simulink model "SpeedControlTest_vDemo_TC"  (Simulink 6.6)
settings: Solver=ode4  SolverMode=SingleTasking  StartTime=0.0  StopTime=252  FixedStep=0.01  RelTol=1e-3
InitFcn:
  | tempomat_para
StopFcn:
  | clear;
values from neighbouring files (symbols this model uses):
  A = 1.9    [tempomat_para.m]
  a_Fzg_max = 2    [tempomat_para.m]
  a_Fzg_min = -2    [tempomat_para.m]
  cw = 0.32    [tempomat_para.m]
  gang = [1 2 3 4]    [tempomat_para.m]
  gang_vec = [1 2 3 4]    [tempomat_para.m]
  i_anteil = 5    [tempomat_para.m]
  i_d = 3.42    [tempomat_para.m]
  i_g = [3.91 2.17 1.37 1.00]    [tempomat_para.m]
  lambda_gang = [1.3 1.25  1.17  1.05]    [tempomat_para.m]
  m_Fzg = 1400    [tempomat_para.m]
  M_mot_max = [130 149 163 170 168 166 162 158 150 139 123 80]    [tempomat_para.m]
  M_mot_min = [0 -40]    [tempomat_para.m]
  n_mot0 = 1000    [tempomat_para.m]
  n_mot_max = 1000:500:6500    [tempomat_para.m]
  n_mot_min = [1000 6500]    [tempomat_para.m]
  p_anteil = 100    [tempomat_para.m]
  r_dyn = 0.28    [tempomat_para.m]
  rho = 1.202    [tempomat_para.m]
  t_sch = 0.2    [tempomat_para.m]
  TI = [block '/TI']    [PSTI_callback.m]
  v_Fzg_ms0 = 0    [tempomat_para.m]
undefined symbols (not defined in the file or in its folder): Drossel_mat, getdatatypespecs
libraries: simulink x113, fzgbib x3
(part 7 of 9)

== system SpeedControlTest_vDemo_TC/Validation Functions/R2 Speed Control velocity restoration time after simple  acceleration or deceleration/after (6 seconds)  |V_Des-V_Vhcl <= 1.4|/PAS1/none - pass - fail/Arbitration ==
  Pass : Inport
  Fail1 : Inport  Port=2
  Fail2 : Inport  Port=3
  Fail3 : Inport  Port=4
  Fail4 : Inport  Port=5
  Delay P F1 F3 : Inport  Port=6
  Delay F2 : Inport  Port=7
  Delay F4 : Inport  Port=8
  Max delay : Inport  Port=9
  Verdict identification : Subsystem
  Verdict selection : Subsystem
  Verdict : Outport
  Delay : Outport  Port=2
  wires:
  Verdict selection/2(Delay) -> Delay/1
  Verdict selection/1(Verdict) -> Verdict/1
  Max delay/1 -> Verdict selection/6(Max delay)
  Verdict identification/2(V2) -> Verdict selection/2(V2)
  Verdict identification/1(V1) -> Verdict selection/1(V1)
  Delay F4/1 -> Verdict selection/5(Delay F4)
  Delay F2/1 -> Verdict selection/4(Delay F2)
  Delay P F1 F3/1 -> Verdict selection/3(Delay P F1 F3)
  Fail4/1 -> Verdict identification/5(Fail4)
  Fail3/1 -> Verdict identification/4(Fail3)
  Fail2/1 -> Verdict identification/3(Fail2)
  Fail1/1 -> Verdict identification/2(Fail1)
  Pass/1 -> Verdict identification/1(Pass)

== system SpeedControlTest_vDemo_TC/Validation Functions/R2 Speed Control velocity restoration time after simple  acceleration or deceleration/after (6 seconds)  |V_Des-V_Vhcl <= 1.4|/PAS1/none - pass - fail/Compute delay ==
  Max Delay : Inport
  R AND : Inport  Port=2
  Clock : Clock
      settings: Decimation=10
  Clock1 : Clock
      settings: Decimation=10
  Divide : Product  Inputs=/*  OutScaling=2^-10
  Hold1 : Subsystem  TreatAsAtomicUnit=on
      mask Display: patch(-0.31+[0.4 0.46 0.46 0.54 0.54 0.6 0.6 0.55 0.55 0.45 0.45 0.4],-0.19+[0.85 0.85 0.95 0.95 0.85 0.85 0.87 0.87 0.96 0.96 0.87 0.87],[0 0 0]);
  SimStepSize : Constant  Value=0.01
  Subtract : Sum  Inputs=-+  OutScaling=2^-10
  Subtract1 : Sum  Inputs=+-  OutScaling=2^-10
  Delay : Outport
  wires:
  Divide/1 -> Delay/1
  Max Delay/1 -> Subtract/1
  SimStepSize/1 -> Divide/1
  Clock/1 -> Hold1/2("    ")
  Subtract/1 -> Subtract1/2
  Subtract1/1 -> Divide/2
  Clock1/1 -> Subtract1/1
  Hold1/1("  ") -> Subtract/2
  R AND/1 -> Hold1/1(" ")

== system SpeedControlTest_vDemo_TC/Validation Functions/R2 Speed Control velocity restoration time after simple  acceleration or deceleration/after (6 seconds)  |V_Des-V_Vhcl <= 1.4|/PAS1/none - pass - fail/Compute delay1 ==
  Max Delay : Inport
  R AND/z : Inport  Port=2
  Add : Sum  OutScaling=2^-10
  Clock : Clock
      settings: Decimation=10
  Clock1 : Clock
      settings: Decimation=10
  Divide : Product  Inputs=/*  OutScaling=2^-10
  Hold1 : Subsystem  TreatAsAtomicUnit=on
      mask Display: patch(-0.31+[0.4 0.46 0.46 0.54 0.54 0.6 0.6 0.55 0.55 0.45 0.45 0.4],-0.19+[0.85 0.85 0.95 0.95 0.85 0.85 0.87 0.87 0.96 0.96 0.87 0.87],[0 0 0]);
  SimStepSize : Constant  Value=0.01
  Subtract : Sum  Inputs=-+  OutScaling=2^-10
  Subtract1 : Sum  Inputs=+-  OutScaling=2^-10
  Unit : Constant
  Delay : Outport
  wires:
  Divide/1 -> Add/2
  Unit/1 -> Add/1
  Max Delay/1 -> Subtract/1
  SimStepSize/1 -> Divide/1
  Clock/1 -> Hold1/2("    ")
  Subtract/1 -> Subtract1/2
  Subtract1/1 -> Divide/2
  Clock1/1 -> Subtract1/1
  Hold1/1("  ") -> Subtract/2
  R AND/z/1 -> Hold1/1(" ")
  Add/1 -> Delay/1

== system SpeedControlTest_vDemo_TC/Validation Functions/R2 Speed Control velocity restoration time after simple  acceleration or deceleration/after (6 seconds)  |V_Des-V_Vhcl <= 1.4|/PAS1/none - pass - fail/Compute delay2 ==
  Max Delay : Inport
  Rp & NOT(Ra) : Inport  Port=2
  Clock : Clock
      settings: Decimation=10
  Clock1 : Clock
      settings: Decimation=10
  Divide : Product  Inputs=/*  OutScaling=2^-10
  Hold1 : Subsystem  TreatAsAtomicUnit=on
      mask Display: patch(-0.31+[0.4 0.46 0.46 0.54 0.54 0.6 0.6 0.55 0.55 0.45 0.45 0.4],-0.19+[0.85 0.85 0.95 0.95 0.85 0.85 0.87 0.87 0.96 0.96 0.87 0.87],[0 0 0]);
  SimStepSize : Constant  Value=0.01
  Subtract : Sum  Inputs=-+  OutScaling=2^-10
  Subtract1 : Sum  Inputs=+-  OutScaling=2^-10
  Delay : Outport
  wires:
  Divide/1 -> Delay/1
  Rp & NOT(Ra)/1 -> Hold1/1(" ")
  Hold1/1("  ") -> Subtract/2
  Clock1/1 -> Subtract1/1
  Subtract1/1 -> Divide/2
  Subtract/1 -> Subtract1/2
  Clock/1 -> Hold1/2("    ")
  SimStepSize/1 -> Divide/1
  Max Delay/1 -> Subtract/1

== system SpeedControlTest_vDemo_TC/Validation Functions/R2 Speed Control velocity restoration time after simple  acceleration or deceleration/after (6 seconds)  |V_Des-V_Vhcl <= 1.4|/PAS1/none - pass - fail/Hold R AND1 ==
  " " : Inport
  "    " : Inport  Port=2
  Memory : Memory  Orientation=left
  Switch : Switch  Criteria=u2 ~= 0
  "  " : Outport
  wires:
  Memory/1 -> Switch/3
  Switch/1 -> Memory/1, "  "/1
  "    "/1 -> Switch/1
  " "/1 -> Switch/2

== system SpeedControlTest_vDemo_TC/Validation Functions/R2 Speed Control velocity restoration time after simple  acceleration or deceleration/after (6 seconds)  |V_Des-V_Vhcl <= 1.4|/PAS1/none - pass - fail/Hold R AND2 ==
  " " : Inport
  "    " : Inport  Port=2
  Memory : Memory  Orientation=left
  Switch : Switch  Criteria=u2 ~= 0
  "  " : Outport
  wires:
  Memory/1 -> Switch/3
  Switch/1 -> Memory/1, "  "/1
  "    "/1 -> Switch/1
  " "/1 -> Switch/2

== system SpeedControlTest_vDemo_TC/Validation Functions/R2 Speed Control velocity restoration time after simple  acceleration or deceleration/after (6 seconds)  |V_Des-V_Vhcl <= 1.4|/PAS1/none - pass - fail/Hold R AND3 ==
  " " : Inport
  "    " : Inport  Port=2
  Memory : Memory  Orientation=left
  Switch : Switch  Criteria=u2 ~= 0
  "  " : Outport
  wires:
  " "/1 -> Switch/2
  "    "/1 -> Switch/1
  Switch/1 -> "  "/1, Memory/1
  Memory/1 -> Switch/3

== system SpeedControlTest_vDemo_TC/Validation Functions/R2 Speed Control velocity restoration time after simple  acceleration or deceleration/after (6 seconds)  |V_Des-V_Vhcl <= 1.4|/PAS1/none - pass - fail/Hold1 ==
  " " : Inport
  "    " : Inport  Port=2
  Memory : Memory  Orientation=left
  Switch : Switch  Criteria=u2 ~= 0
  "  " : Outport
  wires:
  Memory/1 -> Switch/3
  Switch/1 -> Memory/1, "  "/1
  "    "/1 -> Switch/1
  " "/1 -> Switch/2

== system SpeedControlTest_vDemo_TC/Validation Functions/R2 Speed Control velocity restoration time after simple  acceleration or deceleration/after (6 seconds)  |V_Des-V_Vhcl <= 1.4|/PAS1/none - pass - fail/Hold2 ==
  " " : Inport
  "    " : Inport  Port=2
  Memory : Memory  Orientation=left
  Switch : Switch  Criteria=u2 ~= 0
  "  " : Outport
  wires:
  Memory/1 -> Switch/3
  Switch/1 -> Memory/1, "  "/1
  "    "/1 -> Switch/1
  " "/1 -> Switch/2

== system SpeedControlTest_vDemo_TC/Validation Functions/R2 Speed Control velocity restoration time after simple  acceleration or deceleration/after (6 seconds)  |V_Des-V_Vhcl <= 1.4|/PAS1/none - pass - fail/Hold3 ==
  " " : Inport
  "    " : Inport  Port=2
  Memory : Memory  Orientation=left
  Switch : Switch  Criteria=u2 ~= 0
  "  " : Outport
  wires:
  " "/1 -> Switch/2
  "    "/1 -> Switch/1
  Switch/1 -> "  "/1, Memory/1
  Memory/1 -> Switch/3

== system SpeedControlTest_vDemo_TC/Validation Functions/R2 Speed Control velocity restoration time after simple  acceleration or deceleration/after (6 seconds)  |V_Des-V_Vhcl <= 1.4|/PAS1/none - pass - fail/Hold4 ==
  " " : Inport
  "    " : Inport  Port=2
  Memory : Memory  Orientation=left
  Switch : Switch  Criteria=u2 ~= 0
  "  " : Outport
  wires:
  Memory/1 -> Switch/3
  Switch/1 -> Memory/1, "  "/1
  "    "/1 -> Switch/1
  " "/1 -> Switch/2

== system SpeedControlTest_vDemo_TC/Validation Functions/R2 Speed Control velocity restoration time after simple  acceleration or deceleration/after (6 seconds)  |V_Des-V_Vhcl <= 1.4|/PAS1/none - pass - fail/Hold5 ==
  " " : Inport
  "    " : Inport  Port=2
  Memory : Memory  Orientation=left
  Switch : Switch  Criteria=u2 ~= 0
  "  " : Outport
  wires:
  " "/1 -> Switch/2
  "    "/1 -> Switch/1
  Switch/1 -> "  "/1, Memory/1
  Memory/1 -> Switch/3

== system SpeedControlTest_vDemo_TC/Validation Functions/R2 Speed Control velocity restoration time after simple  acceleration or deceleration/after (6 seconds)  |V_Des-V_Vhcl <= 1.4|/PAS2/Delay bus signals/AD delay ==
  In1 : Inport
  Delay : Constant  Value=0
  Integer Delay : S-Function  FunctionName=sfix_udelay  Parameters=samptime,vinit,NumDelays,1,1,0  mask(Integer Delay){vinit=0.0, samptime=-1, NumDelays=15}
      mask prompts: vinit "Initial condition:"; samptime "Sample time:"; NumDelays "Number of delays:"
      mask help: Delay a signal N sample periods.
      mask init:
      | if isempty(NumDelays)
      |    NumDelays = 1;
      | end
      mask Display: fprintf(' %d\nZ   ',-1*(NumDelays))
  Switch : Switch  Criteria=u2 ~= 0
  Out1 : Outport
  wires:
  Switch/1 -> Out1/1
  In1/1 -> Switch/3, Integer Delay/1
  Delay/1 -> Switch/2
  Integer Delay/1 -> Switch/1

== system SpeedControlTest_vDemo_TC/Validation Functions/R2 Speed Control velocity restoration time after simple  acceleration or deceleration/after (6 seconds)  |V_Des-V_Vhcl <= 1.4|/PAS2/Delay bus signals/ELL delay ==
  In1 : Inport
  Delay : Constant  Value=0
  Integer Delay : S-Function  FunctionName=sfix_udelay  Parameters=samptime,vinit,NumDelays,1,1,0  mask(Integer Delay){vinit=0.0, samptime=-1, NumDelays=15}
      mask prompts: vinit "Initial condition:"; samptime "Sample time:"; NumDelays "Number of delays:"
      mask help: Delay a signal N sample periods.
      mask init:
      | if isempty(NumDelays)
      |    NumDelays = 1;
      | end
      mask Display: fprintf(' %d\nZ   ',-1*(NumDelays))
  Switch : Switch  Criteria=u2 ~= 0
  Out1 : Outport
  wires:
  Switch/1 -> Out1/1
  In1/1 -> Switch/3, Integer Delay/1
  Delay/1 -> Switch/2
  Integer Delay/1 -> Switch/1

== system SpeedControlTest_vDemo_TC/Validation Functions/R2 Speed Control velocity restoration time after simple  acceleration or deceleration/after (6 seconds)  |V_Des-V_Vhcl <= 1.4|/PAS2/Delay bus signals/EUL delay ==
  In1 : Inport
  Delay : Constant  Value=0
  Integer Delay : S-Function  FunctionName=sfix_udelay  Parameters=samptime,vinit,NumDelays,1,1,0  mask(Integer Delay){vinit=0.0, samptime=-1, NumDelays=15}
      mask prompts: vinit "Initial condition:"; samptime "Sample time:"; NumDelays "Number of delays:"
      mask help: Delay a signal N sample periods.
      mask init:
      | if isempty(NumDelays)
      |    NumDelays = 1;
      | end
      mask Display: fprintf(' %d\nZ   ',-1*(NumDelays))
  Switch : Switch  Criteria=u2 ~= 0
  Out1 : Outport
  wires:
  Integer Delay/1 -> Switch/1
  Delay/1 -> Switch/2
  In1/1 -> Integer Delay/1, Switch/3
  Switch/1 -> Out1/1

== system SpeedControlTest_vDemo_TC/Validation Functions/R2 Speed Control velocity restoration time after simple  acceleration or deceleration/after (6 seconds)  |V_Des-V_Vhcl <= 1.4|/PAS2/none - pass - fail/Arbitration ==
  Pass : Inport
  Fail1 : Inport  Port=2
  Fail2 : Inport  Port=3
  Fail3 : Inport  Port=4
  Fail4 : Inport  Port=5
  Delay P F1 F3 : Inport  Port=6
  Delay F2 : Inport  Port=7
  Delay F4 : Inport  Port=8
  Max delay : Inport  Port=9
  Verdict identification : Subsystem
  Verdict selection : Subsystem
  Verdict : Outport
  Delay : Outport  Port=2
  wires:
  Verdict selection/2(Delay) -> Delay/1
  Verdict selection/1(Verdict) -> Verdict/1
  Max delay/1 -> Verdict selection/6(Max delay)
  Verdict identification/2(V2) -> Verdict selection/2(V2)
  Verdict identification/1(V1) -> Verdict selection/1(V1)
  Delay F4/1 -> Verdict selection/5(Delay F4)
  Delay F2/1 -> Verdict selection/4(Delay F2)
  Delay P F1 F3/1 -> Verdict selection/3(Delay P F1 F3)
  Fail4/1 -> Verdict identification/5(Fail4)
  Fail3/1 -> Verdict identification/4(Fail3)
  Fail2/1 -> Verdict identification/3(Fail2)
  Fail1/1 -> Verdict identification/2(Fail1)
  Pass/1 -> Verdict identification/1(Pass)

== system SpeedControlTest_vDemo_TC/Validation Functions/R2 Speed Control velocity restoration time after simple  acceleration or deceleration/after (6 seconds)  |V_Des-V_Vhcl <= 1.4|/PAS2/none - pass - fail/Compute delay ==
  Max Delay : Inport
  R AND : Inport  Port=2
  Clock : Clock
      settings: Decimation=10
  Clock1 : Clock
      settings: Decimation=10
  Divide : Product  Inputs=/*  OutScaling=2^-10
  Hold1 : Subsystem  TreatAsAtomicUnit=on
      mask Display: patch(-0.31+[0.4 0.46 0.46 0.54 0.54 0.6 0.6 0.55 0.55 0.45 0.45 0.4],-0.19+[0.85 0.85 0.95 0.95 0.85 0.85 0.87 0.87 0.96 0.96 0.87 0.87],[0 0 0]);
  SimStepSize : Constant  Value=0.01
  Subtract : Sum  Inputs=-+  OutScaling=2^-10
  Subtract1 : Sum  Inputs=+-  OutScaling=2^-10
  Delay : Outport
  wires:
  Divide/1 -> Delay/1
  Max Delay/1 -> Subtract/1
  SimStepSize/1 -> Divide/1
  Clock/1 -> Hold1/2("    ")
  Subtract/1 -> Subtract1/2
  Subtract1/1 -> Divide/2
  Clock1/1 -> Subtract1/1
  Hold1/1("  ") -> Subtract/2
  R AND/1 -> Hold1/1(" ")

== system SpeedControlTest_vDemo_TC/Validation Functions/R2 Speed Control velocity restoration time after simple  acceleration or deceleration/after (6 seconds)  |V_Des-V_Vhcl <= 1.4|/PAS2/none - pass - fail/Compute delay1 ==
  Max Delay : Inport
  R AND/z : Inport  Port=2
  Add : Sum  OutScaling=2^-10
  Clock : Clock
      settings: Decimation=10
  Clock1 : Clock
      settings: Decimation=10
  Divide : Product  Inputs=/*  OutScaling=2^-10
  Hold1 : Subsystem  TreatAsAtomicUnit=on
      mask Display: patch(-0.31+[0.4 0.46 0.46 0.54 0.54 0.6 0.6 0.55 0.55 0.45 0.45 0.4],-0.19+[0.85 0.85 0.95 0.95 0.85 0.85 0.87 0.87 0.96 0.96 0.87 0.87],[0 0 0]);
  SimStepSize : Constant  Value=0.01
  Subtract : Sum  Inputs=-+  OutScaling=2^-10
  Subtract1 : Sum  Inputs=+-  OutScaling=2^-10
  Unit : Constant
  Delay : Outport
  wires:
  Divide/1 -> Add/2
  Unit/1 -> Add/1
  Max Delay/1 -> Subtract/1
  SimStepSize/1 -> Divide/1
  Clock/1 -> Hold1/2("    ")
  Subtract/1 -> Subtract1/2
  Subtract1/1 -> Divide/2
  Clock1/1 -> Subtract1/1
  Hold1/1("  ") -> Subtract/2
  R AND/z/1 -> Hold1/1(" ")
  Add/1 -> Delay/1

== system SpeedControlTest_vDemo_TC/Validation Functions/R2 Speed Control velocity restoration time after simple  acceleration or deceleration/after (6 seconds)  |V_Des-V_Vhcl <= 1.4|/PAS2/none - pass - fail/Compute delay2 ==
  Max Delay : Inport
  Rp & NOT(Ra) : Inport  Port=2
  Clock : Clock
      settings: Decimation=10
  Clock1 : Clock
      settings: Decimation=10
  Divide : Product  Inputs=/*  OutScaling=2^-10
  Hold1 : Subsystem  TreatAsAtomicUnit=on
      mask Display: patch(-0.31+[0.4 0.46 0.46 0.54 0.54 0.6 0.6 0.55 0.55 0.45 0.45 0.4],-0.19+[0.85 0.85 0.95 0.95 0.85 0.85 0.87 0.87 0.96 0.96 0.87 0.87],[0 0 0]);
  SimStepSize : Constant  Value=0.01
  Subtract : Sum  Inputs=-+  OutScaling=2^-10
  Subtract1 : Sum  Inputs=+-  OutScaling=2^-10
  Delay : Outport
  wires:
  Divide/1 -> Delay/1
  Rp & NOT(Ra)/1 -> Hold1/1(" ")
  Hold1/1("  ") -> Subtract/2
  Clock1/1 -> Subtract1/1
  Subtract1/1 -> Divide/2
  Subtract/1 -> Subtract1/2
  Clock/1 -> Hold1/2("    ")
  SimStepSize/1 -> Divide/1
  Max Delay/1 -> Subtract/1

== system SpeedControlTest_vDemo_TC/Validation Functions/R2 Speed Control velocity restoration time after simple  acceleration or deceleration/after (6 seconds)  |V_Des-V_Vhcl <= 1.4|/PAS2/none - pass - fail/Hold R AND1 ==
  " " : Inport
  "    " : Inport  Port=2
  Memory : Memory  Orientation=left
  Switch : Switch  Criteria=u2 ~= 0
  "  " : Outport
  wires:
  Memory/1 -> Switch/3
  Switch/1 -> Memory/1, "  "/1
  "    "/1 -> Switch/1
  " "/1 -> Switch/2

== system SpeedControlTest_vDemo_TC/Validation Functions/R2 Speed Control velocity restoration time after simple  acceleration or deceleration/after (6 seconds)  |V_Des-V_Vhcl <= 1.4|/PAS2/none - pass - fail/Hold R AND2 ==
  " " : Inport
  "    " : Inport  Port=2
  Memory : Memory  Orientation=left
  Switch : Switch  Criteria=u2 ~= 0
  "  " : Outport
  wires:
  Memory/1 -> Switch/3
  Switch/1 -> Memory/1, "  "/1
  "    "/1 -> Switch/1
  " "/1 -> Switch/2

== system SpeedControlTest_vDemo_TC/Validation Functions/R2 Speed Control velocity restoration time after simple  acceleration or deceleration/after (6 seconds)  |V_Des-V_Vhcl <= 1.4|/PAS2/none - pass - fail/Hold R AND3 ==
  " " : Inport
  "    " : Inport  Port=2
  Memory : Memory  Orientation=left
  Switch : Switch  Criteria=u2 ~= 0
  "  " : Outport
  wires:
  " "/1 -> Switch/2
  "    "/1 -> Switch/1
  Switch/1 -> "  "/1, Memory/1
  Memory/1 -> Switch/3

== system SpeedControlTest_vDemo_TC/Validation Functions/R2 Speed Control velocity restoration time after simple  acceleration or deceleration/after (6 seconds)  |V_Des-V_Vhcl <= 1.4|/PAS2/none - pass - fail/Hold1 ==
  " " : Inport
  "    " : Inport  Port=2
  Memory : Memory  Orientation=left
  Switch : Switch  Criteria=u2 ~= 0
  "  " : Outport
  wires:
  Memory/1 -> Switch/3
  Switch/1 -> Memory/1, "  "/1
  "    "/1 -> Switch/1
  " "/1 -> Switch/2

== system SpeedControlTest_vDemo_TC/Validation Functions/R2 Speed Control velocity restoration time after simple  acceleration or deceleration/after (6 seconds)  |V_Des-V_Vhcl <= 1.4|/PAS2/none - pass - fail/Hold2 ==
  " " : Inport
  "    " : Inport  Port=2
  Memory : Memory  Orientation=left
  Switch : Switch  Criteria=u2 ~= 0
  "  " : Outport
  wires:
  Memory/1 -> Switch/3
  Switch/1 -> Memory/1, "  "/1
  "    "/1 -> Switch/1
  " "/1 -> Switch/2

== system SpeedControlTest_vDemo_TC/Validation Functions/R2 Speed Control velocity restoration time after simple  acceleration or deceleration/after (6 seconds)  |V_Des-V_Vhcl <= 1.4|/PAS2/none - pass - fail/Hold3 ==
  " " : Inport
  "    " : Inport  Port=2
  Memory : Memory  Orientation=left
  Switch : Switch  Criteria=u2 ~= 0
  "  " : Outport
  wires:
  " "/1 -> Switch/2
  "    "/1 -> Switch/1
  Switch/1 -> "  "/1, Memory/1
  Memory/1 -> Switch/3

== system SpeedControlTest_vDemo_TC/Validation Functions/R2 Speed Control velocity restoration time after simple  acceleration or deceleration/after (6 seconds)  |V_Des-V_Vhcl <= 1.4|/PAS2/none - pass - fail/Hold4 ==
  " " : Inport
  "    " : Inport  Port=2
  Memory : Memory  Orientation=left
  Switch : Switch  Criteria=u2 ~= 0
  "  " : Outport
  wires:
  Memory/1 -> Switch/3
  Switch/1 -> Memory/1, "  "/1
  "    "/1 -> Switch/1
  " "/1 -> Switch/2

== system SpeedControlTest_vDemo_TC/Validation Functions/R2 Speed Control velocity restoration time after simple  acceleration or deceleration/after (6 seconds)  |V_Des-V_Vhcl <= 1.4|/PAS2/none - pass - fail/Hold5 ==
  " " : Inport
  "    " : Inport  Port=2
  Memory : Memory  Orientation=left
  Switch : Switch  Criteria=u2 ~= 0
  "  " : Outport
  wires:
  " "/1 -> Switch/2
  "    "/1 -> Switch/1
  Switch/1 -> "  "/1, Memory/1
  Memory/1 -> Switch/3

== system SpeedControlTest_vDemo_TC/Validation Functions/R2 Speed Control velocity restoration time after simple  acceleration or deceleration/after (6 seconds)  |V_Des-V_Vhcl <= 1.4|/R = 2/Active for  6s after R=1 /Time since R = 1 ==
  Signal : Inport
  Clock : Clock
      settings: Decimation=10
  Logical Operator : Logic  Operator=NAND  AllPortsSameDT=off  OutDataTypeMode=Boolean
  Logical Operator1 : Logic  Operator=NOT  AllPortsSameDT=off  OutDataTypeMode=Boolean
  Memory : Memory  Orientation=left
  Memory1 : Memory
  R = 1 : Subsystem
  Subtract : Sum  Inputs=-+  OutScaling=2^-10
  Switch : Switch  Criteria=u2 > Threshold
  Trigger : Outport
  Feature : Outport  Port=2
  wires:
  Logical Operator/1 -> Switch/2
  Logical Operator1/1 -> Logical Operator/2
  Memory1/1 -> Logical Operator1/1
  Memory/1 -> Switch/1
  Switch/1 -> Memory/1, Subtract/1
  Clock/1 -> Switch/3, Subtract/2
  Subtract/1 -> Feature/1
  R = 1/1(Out1) -> Memory1/1, Logical Operator/1, Trigger/1
  Signal/1 -> R = 1/1(In1)

== system SpeedControlTest_vDemo_TC/Validation Functions/R1 Speed Control step response/Complete step & CC active + no target & Speed Control active/Complete step detection/Step detection/Active if signals constant for some specified time/Time since signal constant ==
  Signal : Inport
  Clock : Clock
      settings: Decimation=10
  Detect constant : Subsystem  TreatAsAtomicUnit=on  mask(Feature extraction block){RT=0.001}
      mask prompts: RT "Relative tolerance in %"
      mask help: Detect if the signal value is constant (using the last two signal values) allowing for a user-defined relative deviation
      mask CallbackString:
      | if or( (str2double(get_param(gcb,'RT')) < 0), (str2double(get_param(gcb,'RT')) > 100))
      |     error(['Relative tolerance value (' get_param(gcb,'RT') ') out of range. Please give a value between 0 and 100.']);
      | else
      |     set_param([gcb '/Relative tolerance/Relative Tolerance'],'Value',get_param(gcb,'RT'));
      | end
  Logical Operator : Logic  Operator=NAND  AllPortsSameDT=off  OutDataTypeMode=Boolean
  Logical Operator1 : Logic  Operator=NOT  AllPortsSameDT=off  OutDataTypeMode=Boolean
  Memory : Memory  Orientation=left
  Memory1 : Memory
  Subtract : Sum  Inputs=-+  OutScaling=2^-10
  Switch : Switch  Criteria=u2 > Threshold
  Trigger : Outport
  Feature : Outport  Port=2
  wires:
  Logical Operator/1 -> Switch/2
  Logical Operator1/1 -> Logical Operator/2
  Memory1/1 -> Logical Operator1/1
  Memory/1 -> Switch/1
  Switch/1 -> Memory/1, Subtract/1
  Clock/1 -> Switch/3, Subtract/2
  Subtract/1 -> Feature/1
  Detect constant/1(Constant) -> Memory1/1, Logical Operator/1, Trigger/1
  Signal/1 -> Detect constant/1(Signal)

== system SpeedControlTest_vDemo_TC/Validation Functions/R1 Speed Control step response/Complete step & CC active + no target & Speed Control active/Complete step detection/Step detection/Active if signals constant for some specified time/Time since signal constant1 ==
  Signal : Inport
  Clock : Clock
      settings: Decimation=10
  Detect constant : Subsystem  TreatAsAtomicUnit=on  mask(Feature extraction block){RT=0.001}
      mask prompts: RT "Relative tolerance in %"
      mask help: Detect if the signal value is constant (using the last two signal values) allowing for a user-defined relative deviation
      mask CallbackString:
      | if or( (str2double(get_param(gcb,'RT')) < 0), (str2double(get_param(gcb,'RT')) > 100))
      |     error(['Relative tolerance value (' get_param(gcb,'RT') ') out of range. Please give a value between 0 and 100.']);
      | else
      |     set_param([gcb '/Relative tolerance/Relative Tolerance'],'Value',get_param(gcb,'RT'));
      | end
  Logical Operator : Logic  Operator=NAND  AllPortsSameDT=off  OutDataTypeMode=Boolean
  Logical Operator1 : Logic  Operator=NOT  AllPortsSameDT=off  OutDataTypeMode=Boolean
  Memory : Memory  Orientation=left
  Memory1 : Memory
  Subtract : Sum  Inputs=-+  OutScaling=2^-10
  Switch : Switch  Criteria=u2 > Threshold
  Trigger : Outport
  Feature : Outport  Port=2
  wires:
  Signal/1 -> Detect constant/1(Signal)
  Detect constant/1(Constant) -> Trigger/1, Logical Operator/1, Memory1/1
  Subtract/1 -> Feature/1
  Clock/1 -> Subtract/2, Switch/3
  Switch/1 -> Subtract/1, Memory/1
  Memory/1 -> Switch/1
  Memory1/1 -> Logical Operator1/1
  Logical Operator1/1 -> Logical Operator/2
  Logical Operator/1 -> Switch/2

== system SpeedControlTest_vDemo_TC/Validation Functions/R1 Speed Control step response/Complete step & CC active + no target & Speed Control active/Complete step detection/Step detection/Detect constant/Relative tolerance ==
  sig : Inport
  ref : Inport  Port=2
  Abs : Abs
  Abs1 : Abs
  Add : Sum  Inputs=+-  OutScaling=2^-10
  Divide1 : Product  Inputs=**/  OutScaling=2^-10
  Max : Constant  Value=100
  Relational Operator : RelationalOperator  Operator=<=  LogicOutDataTypeMode=Boolean
  Relative Tolerance : Constant  Value=0.0001
  sig == ref : Outport
  wires:
  Abs/1 -> Relational Operator/1
  Add/1 -> Abs/1
  sig/1 -> Add/1
  ref/1 -> Add/2, Abs1/1
  Divide1/1 -> Relational Operator/2
  Max/1 -> Divide1/3
  Relative Tolerance/1 -> Divide1/2
  Relational Operator/1 -> sig == ref/1
  Abs1/1 -> Divide1/1

== system SpeedControlTest_vDemo_TC/Validation Functions/R1 Speed Control step response/Complete step & CC active + no target & Speed Control active/Complete step detection/Step detection reset/Active if signals constant for some specified time/Time since signal constant ==
  Signal : Inport
  Clock : Clock
      settings: Decimation=10
  Detect constant : Subsystem  TreatAsAtomicUnit=on  mask(Feature extraction block){RT=0.0001}
      mask prompts: RT "Relative tolerance in %"
      mask help: Detect if the signal value is constant (using the last two signal values) allowing for a user-defined relative deviation
      mask CallbackString:
      | if or( (str2double(get_param(gcb,'RT')) < 0), (str2double(get_param(gcb,'RT')) > 100))
      |     error(['Relative tolerance value (' get_param(gcb,'RT') ') out of range. Please give a value between 0 and 100.']);
      | else
      |     set_param([gcb '/Relative tolerance/Relative Tolerance'],'Value',get_param(gcb,'RT'));
      | end
  Logical Operator : Logic  Operator=NAND  AllPortsSameDT=off  OutDataTypeMode=Boolean
  Logical Operator1 : Logic  Operator=NOT  AllPortsSameDT=off  OutDataTypeMode=Boolean
  Memory : Memory  Orientation=left
  Memory1 : Memory
  Subtract : Sum  Inputs=-+  OutScaling=2^-10
  Switch : Switch  Criteria=u2 > Threshold
  Trigger : Outport
  Feature : Outport  Port=2
  wires:
  Signal/1 -> Detect constant/1(Signal)
  Detect constant/1(Constant) -> Trigger/1, Logical Operator/1, Memory1/1
  Subtract/1 -> Feature/1
  Clock/1 -> Subtract/2, Switch/3
  Switch/1 -> Subtract/1, Memory/1
  Memory/1 -> Switch/1
  Memory1/1 -> Logical Operator1/1
  Logical Operator1/1 -> Logical Operator/2
  Logical Operator/1 -> Switch/2

== system SpeedControlTest_vDemo_TC/Validation Functions/R1 Speed Control step response/Complete step & CC active + no target & Speed Control active/Complete step detection/Step detection reset/Active if signals constant for some specified time/Time since signal constant1 ==
  Signal : Inport
  Clock : Clock
      settings: Decimation=10
  Detect constant : Subsystem  TreatAsAtomicUnit=on  mask(Feature extraction block){RT=0.0001}
      mask prompts: RT "Relative tolerance in %"
      mask help: Detect if the signal value is constant (using the last two signal values) allowing for a user-defined relative deviation
      mask CallbackString:
      | if or( (str2double(get_param(gcb,'RT')) < 0), (str2double(get_param(gcb,'RT')) > 100))
      |     error(['Relative tolerance value (' get_param(gcb,'RT') ') out of range. Please give a value between 0 and 100.']);
      | else
      |     set_param([gcb '/Relative tolerance/Relative Tolerance'],'Value',get_param(gcb,'RT'));
      | end
  Logical Operator : Logic  Operator=NAND  AllPortsSameDT=off  OutDataTypeMode=Boolean
  Logical Operator1 : Logic  Operator=NOT  AllPortsSameDT=off  OutDataTypeMode=Boolean
  Memory : Memory  Orientation=left
  Memory1 : Memory
  Subtract : Sum  Inputs=-+  OutScaling=2^-10
  Switch : Switch  Criteria=u2 > Threshold
  Trigger : Outport
  Feature : Outport  Port=2
  wires:
  Logical Operator/1 -> Switch/2
  Logical Operator1/1 -> Logical Operator/2
  Memory1/1 -> Logical Operator1/1
  Memory/1 -> Switch/1
  Switch/1 -> Memory/1, Subtract/1
  Clock/1 -> Switch/3, Subtract/2
  Subtract/1 -> Feature/1
  Detect constant/1(Constant) -> Memory1/1, Logical Operator/1, Trigger/1
  Signal/1 -> Detect constant/1(Signal)

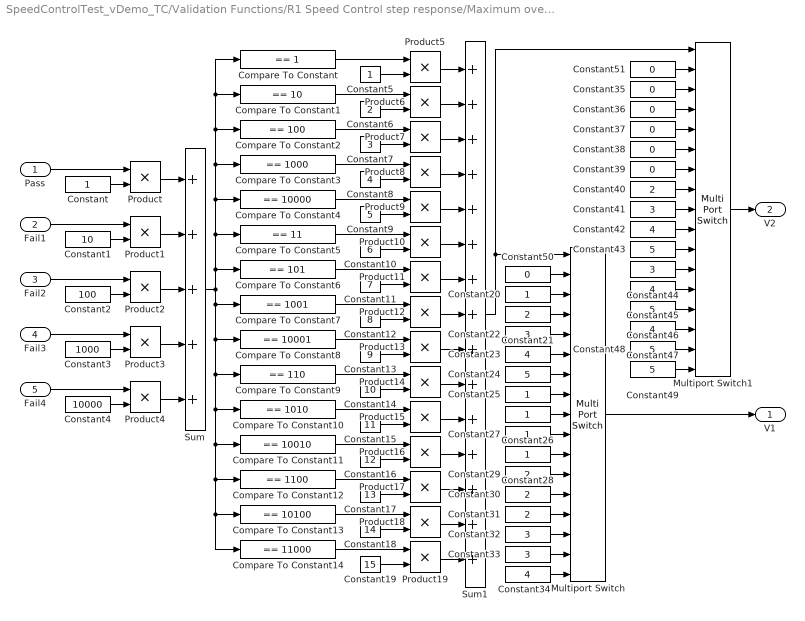
== system SpeedControlTest_vDemo_TC/Validation Functions/R1 Speed Control step response/Maximum overshoot < 5 &  Steady state error < 5/PAS/none - pass - fail/Arbitration/Verdict identification ==
  Pass : Inport
  Fail1 : Inport  Port=2
  Fail2 : Inport  Port=3
  Fail3 : Inport  Port=4
  Fail4 : Inport  Port=5
  Compare To Constant : simulink/Logic and Bit Operations/Compare To Constant  SystemSampleTime=-1  relop===  const=1  LogicOutDataTypeMode=uint8  ZeroCross=off
  Compare To Constant1 : simulink/Logic and Bit Operations/Compare To Constant  SystemSampleTime=-1  relop===  const=10  LogicOutDataTypeMode=uint8  ZeroCross=off
  Compare To Constant10 : simulink/Logic and Bit Operations/Compare To Constant  SystemSampleTime=-1  relop===  const=1010  LogicOutDataTypeMode=uint8  ZeroCross=off
  Compare To Constant11 : simulink/Logic and Bit Operations/Compare To Constant  SystemSampleTime=-1  relop===  const=10010  LogicOutDataTypeMode=uint8  ZeroCross=off
  Compare To Constant12 : simulink/Logic and Bit Operations/Compare To Constant  SystemSampleTime=-1  relop===  const=1100  LogicOutDataTypeMode=uint8  ZeroCross=off
  Compare To Constant13 : simulink/Logic and Bit Operations/Compare To Constant  SystemSampleTime=-1  relop===  const=10100  LogicOutDataTypeMode=uint8  ZeroCross=off
  Compare To Constant14 : simulink/Logic and Bit Operations/Compare To Constant  SystemSampleTime=-1  relop===  const=11000  LogicOutDataTypeMode=uint8  ZeroCross=off
  Compare To Constant2 : simulink/Logic and Bit Operations/Compare To Constant  SystemSampleTime=-1  relop===  const=100  LogicOutDataTypeMode=uint8  ZeroCross=off
  Compare To Constant3 : simulink/Logic and Bit Operations/Compare To Constant  SystemSampleTime=-1  relop===  const=1000  LogicOutDataTypeMode=uint8  ZeroCross=off
  Compare To Constant4 : simulink/Logic and Bit Operations/Compare To Constant  SystemSampleTime=-1  relop===  const=10000  LogicOutDataTypeMode=uint8  ZeroCross=off
  Compare To Constant5 : simulink/Logic and Bit Operations/Compare To Constant  SystemSampleTime=-1  relop===  const=11  LogicOutDataTypeMode=uint8  ZeroCross=off
  Compare To Constant6 : simulink/Logic and Bit Operations/Compare To Constant  SystemSampleTime=-1  relop===  const=101  LogicOutDataTypeMode=uint8  ZeroCross=off
  Compare To Constant7 : simulink/Logic and Bit Operations/Compare To Constant  SystemSampleTime=-1  relop===  const=1001  LogicOutDataTypeMode=uint8  ZeroCross=off
  Compare To Constant8 : simulink/Logic and Bit Operations/Compare To Constant  SystemSampleTime=-1  relop===  const=10001  LogicOutDataTypeMode=uint8  ZeroCross=off
  Compare To Constant9 : simulink/Logic and Bit Operations/Compare To Constant  SystemSampleTime=-1  relop===  const=110  LogicOutDataTypeMode=uint8  ZeroCross=off
  Constant{,5,20,25..28} (7 alike) : Constant
  Constant1 : Constant  Value=10
  Constant10 : Constant  Value=6
  Constant11 : Constant  Value=7
  Constant12 : Constant  Value=8
  Constant13 : Constant  Value=9
  Constant14 : Constant  Value=10
  Constant15 : Constant  Value=11
  Constant16 : Constant  Value=12
  Constant17 : Constant  Value=13
  Constant18 : Constant  Value=14
  Constant19 : Constant  Value=15
  Constant2 : Constant  Value=100
  Constant{6,21,29..31,40} (6 alike) : Constant  Value=2
  Constant{7,22,32..33,41,44} (6 alike) : Constant  Value=3
  Constant{8,23,34,42,45,47} (6 alike) : Constant  Value=4
  Constant{9,24,43,46,48..49} (6 alike) : Constant  Value=5
  Constant3 : Constant  Value=1000
  Constant{35..39,50..51} (7 alike) : Constant  Value=0
  Constant4 : Constant  Value=10000
  Multiport Switch : MultiPortSwitch  Inputs=16  zeroidx=on
  Multiport Switch1 : MultiPortSwitch  Inputs=16  zeroidx=on
  Product{,1..19} (20 alike) : Product  RndMeth=Zero
  Sum : Sum  Inputs=+++++
  Sum1 : Sum  Inputs=+++++++++++++++
  V1 : Outport
  V2 : Outport  Port=2
  wires:
  Constant51/1 -> Multiport Switch1/2
  Constant34/1 -> Multiport Switch/17
  Constant33/1 -> Multiport Switch/16
  Constant32/1 -> Multiport Switch/15
  Constant31/1 -> Multiport Switch/14
  Constant30/1 -> Multiport Switch/13
  Constant29/1 -> Multiport Switch/12
  Constant28/1 -> Multiport Switch/11
  Constant27/1 -> Multiport Switch/10
  Constant26/1 -> Multiport Switch/9
  Constant25/1 -> Multiport Switch/8
  Constant24/1 -> Multiport Switch/7
  Constant23/1 -> Multiport Switch/6
  Constant22/1 -> Multiport Switch/5
  Constant21/1 -> Multiport Switch/4
  Constant20/1 -> Multiport Switch/3
  Constant50/1 -> Multiport Switch/2
  Product19/1 -> Sum1/15
  Product18/1 -> Sum1/14
  Product17/1 -> Sum1/13
  Product16/1 -> Sum1/12
  Product15/1 -> Sum1/11
  Product14/1 -> Sum1/10
  Product13/1 -> Sum1/9
  Product12/1 -> Sum1/8
  Product11/1 -> Sum1/7
  Product10/1 -> Sum1/6
  Product9/1 -> Sum1/5
  Product8/1 -> Sum1/4
  Product7/1 -> Sum1/3
  Product6/1 -> Sum1/2
  Product5/1 -> Sum1/1
  Multiport Switch1/1 -> V2/1
  Constant49/1 -> Multiport Switch1/17
  Constant48/1 -> Multiport Switch1/16
  Constant47/1 -> Multiport Switch1/15
  Constant46/1 -> Multiport Switch1/14
  Constant45/1 -> Multiport Switch1/13
  Constant44/1 -> Multiport Switch1/12
  Constant43/1 -> Multiport Switch1/11
  Constant42/1 -> Multiport Switch1/10
  Constant41/1 -> Multiport Switch1/9
  Constant40/1 -> Multiport Switch1/8
  Constant39/1 -> Multiport Switch1/7
  Constant38/1 -> Multiport Switch1/6
  Constant37/1 -> Multiport Switch1/5
  Constant36/1 -> Multiport Switch1/4
  Constant35/1 -> Multiport Switch1/3
  Sum1/1 -> Multiport Switch1/1, Multiport Switch/1
  Multiport Switch/1 -> V1/1
  Sum/1 -> Compare To Constant7/1, Compare To Constant13/1, Compare To Constant14/1, Compare To Constant12/1, Compare To Constant11/1, Compare To Constant10/1, Compare To Constant9/1, Compare To Constant8/1, Compare To Constant/1, Compare To Constant1/1, Compare To Constant2/1, Compare To Constant3/1, Compare To Constant4/1, Compare To Constant5/1, Compare To Constant6/1
  Compare To Constant14/1 -> Product19/1
  Constant19/1 -> Product19/2
  Compare To Constant13/1 -> Product18/1
  Constant18/1 -> Product18/2
  Compare To Constant12/1 -> Product17/1
  Constant17/1 -> Product17/2
  Compare To Constant11/1 -> Product16/1
  Constant16/1 -> Product16/2
  Compare To Constant10/1 -> Product15/1
  Constant15/1 -> Product15/2
  Compare To Constant9/1 -> Product14/1
  Constant14/1 -> Product14/2
  Compare To Constant8/1 -> Product13/1
  Constant13/1 -> Product13/2
  Compare To Constant7/1 -> Product12/1
  Constant12/1 -> Product12/2
  Compare To Constant6/1 -> Product11/1
  Constant11/1 -> Product11/2
  Compare To Constant5/1 -> Product10/1
  Constant10/1 -> Product10/2
  Compare To Constant4/1 -> Product9/1
  Constant9/1 -> Product9/2
  Compare To Constant3/1 -> Product8/1
  Compare To Constant2/1 -> Product7/1
  Constant8/1 -> Product8/2
  Constant7/1 -> Product7/2
  Compare To Constant1/1 -> Product6/1
  Constant6/1 -> Product6/2
  Constant5/1 -> Product5/2
  Compare To Constant/1 -> Product5/1
  Product4/1 -> Sum/5
  Product3/1 -> Sum/4
  Product2/1 -> Sum/3
  Product1/1 -> Sum/2
  Product/1 -> Sum/1
  Constant/1 -> Product/2
  Constant1/1 -> Product1/2
  Constant2/1 -> Product2/2
  Constant4/1 -> Product4/2
  Constant3/1 -> Product3/2
  Fail4/1 -> Product4/1
  Fail3/1 -> Product3/1
  Fail2/1 -> Product2/1
  Fail1/1 -> Product1/1
  Pass/1 -> Product/1

== system SpeedControlTest_vDemo_TC/Validation Functions/R1 Speed Control step response/Maximum overshoot < 5 &  Steady state error < 5/PAS/none - pass - fail/Arbitration/Verdict selection ==
  V1 : Inport
  V2 : Inport  Port=2
  Delay P F1 F3 : Inport  Port=3
  Delay F2 : Inport  Port=4
  Delay F4 : Inport  Port=5
  Max delay : Inport  Port=6
  Compare To Zero1 : simulink/Logic and Bit Operations/Compare To Zero  SystemSampleTime=-1  relop=~=  LogicOutDataTypeMode=boolean  ZeroCross=off
  Constant{2..4,39} (4 alike) : Constant  Value=0
  Constant35 : Constant
  Constant40 : Constant  Value=2
  Memory : Memory
  Memory1 : Memory
  Multiport Switch1 : MultiPortSwitch  Inputs=6  zeroidx=on
  Multiport Switch2 : MultiPortSwitch  Inputs=6  zeroidx=on
  Multiport Switch4 : MultiPortSwitch  Inputs=6  zeroidx=on
  Sum : Sum
  Switch : Switch  Criteria=u2 ~= 0
  Switch1 : Switch  Criteria=u2 ~= 0
  Switch2 : Switch  Criteria=u2 ~= 0
  Unit : Constant
  Verdict : Outport
  Delay : Outport  Port=2
  wires:
  Switch2/1 -> Multiport Switch4/1, Memory/1
  Unit/1 -> Sum/1
  Memory1/1 -> Sum/2
  Sum/1 -> Switch1/1
  Multiport Switch4/1 -> Memory1/1
  Multiport Switch2/1 -> Switch1/3
  Switch1/1 -> Delay/1
  Switch/1 -> Multiport Switch1/1
  Compare To Zero1/1 -> Switch2/2, Switch1/2, Switch/2
  Memory/1 -> Switch/1, Compare To Zero1/1
  Delay F4/1 -> Multiport Switch4/7, Multiport Switch2/7
  Delay F2/1 -> Multiport Switch4/5, Multiport Switch2/5
  Delay P F1 F3/1 -> Multiport Switch4/3, Multiport Switch4/4, Multiport Switch4/6, Multiport Switch2/4, Multiport Switch2/6, Multiport Switch2/3
  Max delay/1 -> Multiport Switch4/2, Multiport Switch2/2
  V1/1 -> Switch2/1, Switch/3, Multiport Switch2/1
  V2/1 -> Switch2/3
  Constant40/1 -> Multiport Switch1/2
  Constant35/1 -> Multiport Switch1/3
  Constant4/1 -> Multiport Switch1/4
  Constant3/1 -> Multiport Switch1/5
  Constant2/1 -> Multiport Switch1/6
  Constant39/1 -> Multiport Switch1/7
  Multiport Switch1/1 -> Verdict/1

== system SpeedControlTest_vDemo_TC/Validation Functions/R1 Speed Control step response/Maximum overshoot < 5 &  Steady state error < 5/PAS/none - pass - fail/Compute delay/Hold1 ==
  " " : Inport
  "    " : Inport  Port=2
  Memory : Memory  Orientation=left
  Switch : Switch  Criteria=u2 ~= 0
  "  " : Outport
  wires:
  " "/1 -> Switch/2
  "    "/1 -> Switch/1
  Switch/1 -> "  "/1, Memory/1
  Memory/1 -> Switch/3

== system SpeedControlTest_vDemo_TC/Validation Functions/R1 Speed Control step response/Maximum overshoot < 5 &  Steady state error < 5/PAS/none - pass - fail/Compute delay1/Hold1 ==
  " " : Inport
  "    " : Inport  Port=2
  Memory : Memory  Orientation=left
  Switch : Switch  Criteria=u2 ~= 0
  "  " : Outport
  wires:
  " "/1 -> Switch/2
  "    "/1 -> Switch/1
  Switch/1 -> "  "/1, Memory/1
  Memory/1 -> Switch/3

== system SpeedControlTest_vDemo_TC/Validation Functions/R1 Speed Control step response/Maximum overshoot < 5 &  Steady state error < 5/PAS/none - pass - fail/Compute delay2/Hold1 ==
  " " : Inport
  "    " : Inport  Port=2
  Memory : Memory  Orientation=left
  Switch : Switch  Criteria=u2 ~= 0
  "  " : Outport
  wires:
  Memory/1 -> Switch/3
  Switch/1 -> Memory/1, "  "/1
  "    "/1 -> Switch/1
  " "/1 -> Switch/2

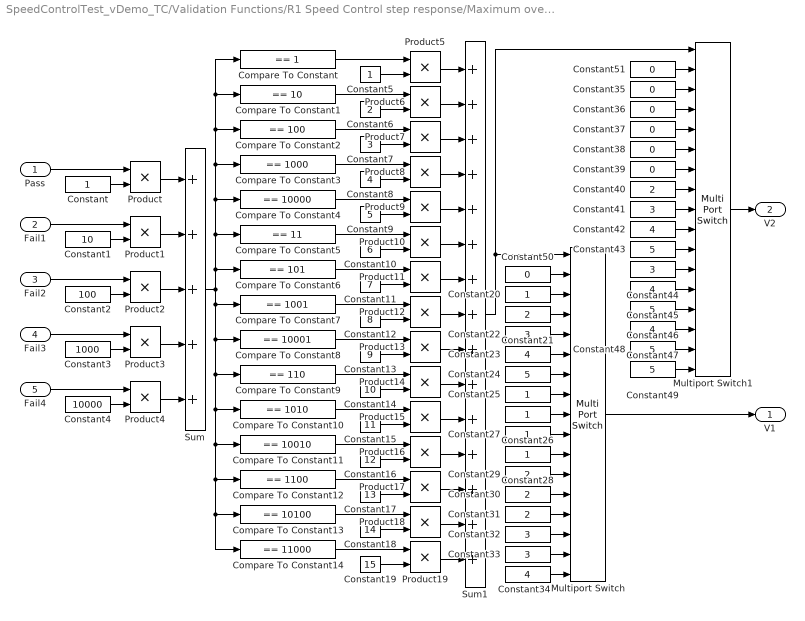
== system SpeedControlTest_vDemo_TC/Validation Functions/R1 Speed Control step response/Maximum overshoot < 5 &  Steady state error < 5/PAS1/none - pass - fail/Arbitration/Verdict identification ==
  Pass : Inport
  Fail1 : Inport  Port=2
  Fail2 : Inport  Port=3
  Fail3 : Inport  Port=4
  Fail4 : Inport  Port=5
  Compare To Constant : simulink/Logic and Bit Operations/Compare To Constant  SystemSampleTime=-1  relop===  const=1  LogicOutDataTypeMode=uint8  ZeroCross=off
  Compare To Constant1 : simulink/Logic and Bit Operations/Compare To Constant  SystemSampleTime=-1  relop===  const=10  LogicOutDataTypeMode=uint8  ZeroCross=off
  Compare To Constant10 : simulink/Logic and Bit Operations/Compare To Constant  SystemSampleTime=-1  relop===  const=1010  LogicOutDataTypeMode=uint8  ZeroCross=off
  Compare To Constant11 : simulink/Logic and Bit Operations/Compare To Constant  SystemSampleTime=-1  relop===  const=10010  LogicOutDataTypeMode=uint8  ZeroCross=off
  Compare To Constant12 : simulink/Logic and Bit Operations/Compare To Constant  SystemSampleTime=-1  relop===  const=1100  LogicOutDataTypeMode=uint8  ZeroCross=off
  Compare To Constant13 : simulink/Logic and Bit Operations/Compare To Constant  SystemSampleTime=-1  relop===  const=10100  LogicOutDataTypeMode=uint8  ZeroCross=off
  Compare To Constant14 : simulink/Logic and Bit Operations/Compare To Constant  SystemSampleTime=-1  relop===  const=11000  LogicOutDataTypeMode=uint8  ZeroCross=off
  Compare To Constant2 : simulink/Logic and Bit Operations/Compare To Constant  SystemSampleTime=-1  relop===  const=100  LogicOutDataTypeMode=uint8  ZeroCross=off
  Compare To Constant3 : simulink/Logic and Bit Operations/Compare To Constant  SystemSampleTime=-1  relop===  const=1000  LogicOutDataTypeMode=uint8  ZeroCross=off
  Compare To Constant4 : simulink/Logic and Bit Operations/Compare To Constant  SystemSampleTime=-1  relop===  const=10000  LogicOutDataTypeMode=uint8  ZeroCross=off
  Compare To Constant5 : simulink/Logic and Bit Operations/Compare To Constant  SystemSampleTime=-1  relop===  const=11  LogicOutDataTypeMode=uint8  ZeroCross=off
  Compare To Constant6 : simulink/Logic and Bit Operations/Compare To Constant  SystemSampleTime=-1  relop===  const=101  LogicOutDataTypeMode=uint8  ZeroCross=off
  Compare To Constant7 : simulink/Logic and Bit Operations/Compare To Constant  SystemSampleTime=-1  relop===  const=1001  LogicOutDataTypeMode=uint8  ZeroCross=off
  Compare To Constant8 : simulink/Logic and Bit Operations/Compare To Constant  SystemSampleTime=-1  relop===  const=10001  LogicOutDataTypeMode=uint8  ZeroCross=off
  Compare To Constant9 : simulink/Logic and Bit Operations/Compare To Constant  SystemSampleTime=-1  relop===  const=110  LogicOutDataTypeMode=uint8  ZeroCross=off
  Constant{,5,20,25..28} (7 alike) : Constant
  Constant1 : Constant  Value=10
  Constant10 : Constant  Value=6
  Constant11 : Constant  Value=7
  Constant12 : Constant  Value=8
  Constant13 : Constant  Value=9
  Constant14 : Constant  Value=10
  Constant15 : Constant  Value=11
  Constant16 : Constant  Value=12
  Constant17 : Constant  Value=13
  Constant18 : Constant  Value=14
  Constant19 : Constant  Value=15
  Constant2 : Constant  Value=100
  Constant{6,21,29..31,40} (6 alike) : Constant  Value=2
  Constant{7,22,32..33,41,44} (6 alike) : Constant  Value=3
  Constant{8,23,34,42,45,47} (6 alike) : Constant  Value=4
  Constant{9,24,43,46,48..49} (6 alike) : Constant  Value=5
  Constant3 : Constant  Value=1000
  Constant{35..39,50..51} (7 alike) : Constant  Value=0
  Constant4 : Constant  Value=10000
  Multiport Switch : MultiPortSwitch  Inputs=16  zeroidx=on
  Multiport Switch1 : MultiPortSwitch  Inputs=16  zeroidx=on
  Product{,1..19} (20 alike) : Product  RndMeth=Zero
  Sum : Sum  Inputs=+++++
  Sum1 : Sum  Inputs=+++++++++++++++
  V1 : Outport
  V2 : Outport  Port=2
  wires:
  Pass/1 -> Product/1
  Fail1/1 -> Product1/1
  Fail2/1 -> Product2/1
  Fail3/1 -> Product3/1
  Fail4/1 -> Product4/1
  Constant3/1 -> Product3/2
  Constant4/1 -> Product4/2
  Constant2/1 -> Product2/2
  Constant1/1 -> Product1/2
  Constant/1 -> Product/2
  Product/1 -> Sum/1
  Product1/1 -> Sum/2
  Product2/1 -> Sum/3
  Product3/1 -> Sum/4
  Product4/1 -> Sum/5
  Compare To Constant/1 -> Product5/1
  Constant5/1 -> Product5/2
  Constant6/1 -> Product6/2
  Compare To Constant1/1 -> Product6/1
  Constant7/1 -> Product7/2
  Constant8/1 -> Product8/2
  Compare To Constant2/1 -> Product7/1
  Compare To Constant3/1 -> Product8/1
  Constant9/1 -> Product9/2
  Compare To Constant4/1 -> Product9/1
  Constant10/1 -> Product10/2
  Compare To Constant5/1 -> Product10/1
  Constant11/1 -> Product11/2
  Compare To Constant6/1 -> Product11/1
  Constant12/1 -> Product12/2
  Compare To Constant7/1 -> Product12/1
  Constant13/1 -> Product13/2
  Compare To Constant8/1 -> Product13/1
  Constant14/1 -> Product14/2
  Compare To Constant9/1 -> Product14/1
  Constant15/1 -> Product15/2
  Compare To Constant10/1 -> Product15/1
  Constant16/1 -> Product16/2
  Compare To Constant11/1 -> Product16/1
  Constant17/1 -> Product17/2
  Compare To Constant12/1 -> Product17/1
  Constant18/1 -> Product18/2
  Compare To Constant13/1 -> Product18/1
  Constant19/1 -> Product19/2
  Compare To Constant14/1 -> Product19/1
  Sum/1 -> Compare To Constant6/1, Compare To Constant5/1, Compare To Constant4/1, Compare To Constant3/1, Compare To Constant2/1, Compare To Constant1/1, Compare To Constant/1, Compare To Constant8/1, Compare To Constant9/1, Compare To Constant10/1, Compare To Constant11/1, Compare To Constant12/1, Compare To Constant14/1, Compare To Constant13/1, Compare To Constant7/1
  Multiport Switch/1 -> V1/1
  Sum1/1 -> Multiport Switch/1, Multiport Switch1/1
  Constant35/1 -> Multiport Switch1/3
  Constant36/1 -> Multiport Switch1/4
  Constant37/1 -> Multiport Switch1/5
  Constant38/1 -> Multiport Switch1/6
  Constant39/1 -> Multiport Switch1/7
  Constant40/1 -> Multiport Switch1/8
  Constant41/1 -> Multiport Switch1/9
  Constant42/1 -> Multiport Switch1/10
  Constant43/1 -> Multiport Switch1/11
  Constant44/1 -> Multiport Switch1/12
  Constant45/1 -> Multiport Switch1/13
  Constant46/1 -> Multiport Switch1/14
  Constant47/1 -> Multiport Switch1/15
  Constant48/1 -> Multiport Switch1/16
  Constant49/1 -> Multiport Switch1/17
  Multiport Switch1/1 -> V2/1
  Product5/1 -> Sum1/1
  Product6/1 -> Sum1/2
  Product7/1 -> Sum1/3
  Product8/1 -> Sum1/4
  Product9/1 -> Sum1/5
  Product10/1 -> Sum1/6
  Product11/1 -> Sum1/7
  Product12/1 -> Sum1/8
  Product13/1 -> Sum1/9
  Product14/1 -> Sum1/10
  Product15/1 -> Sum1/11
  Product16/1 -> Sum1/12
  Product17/1 -> Sum1/13
  Product18/1 -> Sum1/14
  Product19/1 -> Sum1/15
  Constant50/1 -> Multiport Switch/2
  Constant20/1 -> Multiport Switch/3
  Constant21/1 -> Multiport Switch/4
  Constant22/1 -> Multiport Switch/5
  Constant23/1 -> Multiport Switch/6
  Constant24/1 -> Multiport Switch/7
  Constant25/1 -> Multiport Switch/8
  Constant26/1 -> Multiport Switch/9
  Constant27/1 -> Multiport Switch/10
  Constant28/1 -> Multiport Switch/11
  Constant29/1 -> Multiport Switch/12
  Constant30/1 -> Multiport Switch/13
  Constant31/1 -> Multiport Switch/14
  Constant32/1 -> Multiport Switch/15
  Constant33/1 -> Multiport Switch/16
  Constant34/1 -> Multiport Switch/17
  Constant51/1 -> Multiport Switch1/2

== system SpeedControlTest_vDemo_TC/Validation Functions/R1 Speed Control step response/Maximum overshoot < 5 &  Steady state error < 5/PAS1/none - pass - fail/Arbitration/Verdict selection ==
  V1 : Inport
  V2 : Inport  Port=2
  Delay P F1 F3 : Inport  Port=3
  Delay F2 : Inport  Port=4
  Delay F4 : Inport  Port=5
  Max delay : Inport  Port=6
  Compare To Zero1 : simulink/Logic and Bit Operations/Compare To Zero  SystemSampleTime=-1  relop=~=  LogicOutDataTypeMode=boolean  ZeroCross=off
  Constant{2..4,39} (4 alike) : Constant  Value=0
  Constant35 : Constant
  Constant40 : Constant  Value=2
  Memory : Memory
  Memory1 : Memory
  Multiport Switch1 : MultiPortSwitch  Inputs=6  zeroidx=on
  Multiport Switch2 : MultiPortSwitch  Inputs=6  zeroidx=on
  Multiport Switch4 : MultiPortSwitch  Inputs=6  zeroidx=on
  Sum : Sum
  Switch : Switch  Criteria=u2 ~= 0
  Switch1 : Switch  Criteria=u2 ~= 0
  Switch2 : Switch  Criteria=u2 ~= 0
  Unit : Constant
  Verdict : Outport
  Delay : Outport  Port=2
  wires:
  Multiport Switch1/1 -> Verdict/1
  Constant39/1 -> Multiport Switch1/7
  Constant2/1 -> Multiport Switch1/6
  Constant3/1 -> Multiport Switch1/5
  Constant4/1 -> Multiport Switch1/4
  Constant35/1 -> Multiport Switch1/3
  Constant40/1 -> Multiport Switch1/2
  V2/1 -> Switch2/3
  V1/1 -> Multiport Switch2/1, Switch/3, Switch2/1
  Max delay/1 -> Multiport Switch2/2, Multiport Switch4/2
  Delay P F1 F3/1 -> Multiport Switch2/3, Multiport Switch2/6, Multiport Switch2/4, Multiport Switch4/6, Multiport Switch4/4, Multiport Switch4/3
  Delay F2/1 -> Multiport Switch2/5, Multiport Switch4/5
  Delay F4/1 -> Multiport Switch2/7, Multiport Switch4/7
  Memory/1 -> Compare To Zero1/1, Switch/1
  Compare To Zero1/1 -> Switch/2, Switch1/2, Switch2/2
  Switch/1 -> Multiport Switch1/1
  Switch1/1 -> Delay/1
  Multiport Switch2/1 -> Switch1/3
  Multiport Switch4/1 -> Memory1/1
  Sum/1 -> Switch1/1
  Memory1/1 -> Sum/2
  Unit/1 -> Sum/1
  Switch2/1 -> Memory/1, Multiport Switch4/1

== system SpeedControlTest_vDemo_TC/Validation Functions/R1 Speed Control step response/Maximum overshoot < 5 &  Steady state error < 5/PAS1/none - pass - fail/Compute delay/Hold1 ==
  " " : Inport
  "    " : Inport  Port=2
  Memory : Memory  Orientation=left
  Switch : Switch  Criteria=u2 ~= 0
  "  " : Outport
  wires:
  Memory/1 -> Switch/3
  Switch/1 -> Memory/1, "  "/1
  "    "/1 -> Switch/1
  " "/1 -> Switch/2

== system SpeedControlTest_vDemo_TC/Validation Functions/R1 Speed Control step response/Maximum overshoot < 5 &  Steady state error < 5/PAS1/none - pass - fail/Compute delay1/Hold1 ==
  " " : Inport
  "    " : Inport  Port=2
  Memory : Memory  Orientation=left
  Switch : Switch  Criteria=u2 ~= 0
  "  " : Outport
  wires:
  Memory/1 -> Switch/3
  Switch/1 -> Memory/1, "  "/1
  "    "/1 -> Switch/1
  " "/1 -> Switch/2

== system SpeedControlTest_vDemo_TC/Validation Functions/R1 Speed Control step response/Maximum overshoot < 5 &  Steady state error < 5/PAS1/none - pass - fail/Compute delay2/Hold1 ==
  " " : Inport
  "    " : Inport  Port=2
  Memory : Memory  Orientation=left
  Switch : Switch  Criteria=u2 ~= 0
  "  " : Outport
  wires:
  " "/1 -> Switch/2
  "    "/1 -> Switch/1
  Switch/1 -> "  "/1, Memory/1
  Memory/1 -> Switch/3
